simulink model "sim4"  (R2024a)
settings: Solver=FixedStepAuto  StartTime=0.0  StopTime=10.0  FixedStep=1  RelTol=1e-3
settings Model: Creator=alexe  LastModifiedBy=alexe

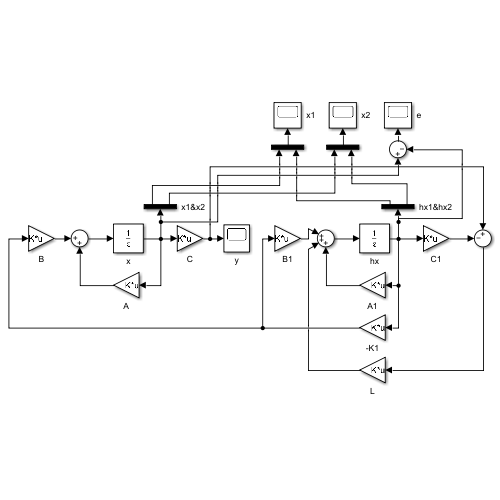
[thumbnail: Simulink's stored preview of the top-level diagram]
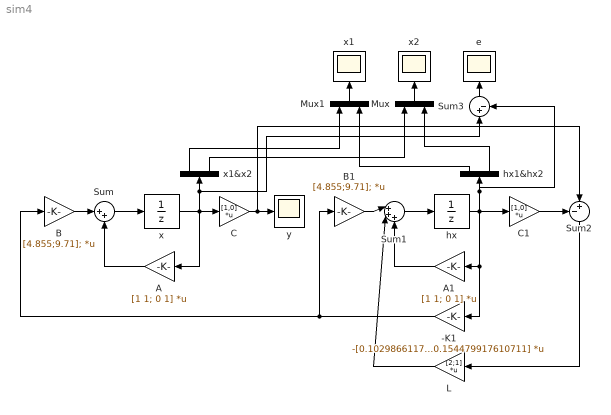
== system sim4 ==
  -K1 : Gain  Gain=-[0.102986611740474,0.154479917610711]  Multiplication=Matrix(K*u)
  A : Gain  Gain=[1 1; 0 1]  Multiplication=Matrix(K*u)
  A1 : Gain  Gain=[1 1; 0 1]  Multiplication=Matrix(K*u)
  B : Gain  Gain=[4.855;9.71];  Multiplication=Matrix(K*u)
  B1 : Gain  Gain=[4.855;9.71];  Multiplication=Matrix(K*u)
  C : Gain  Gain=[1,0]  Multiplication=Matrix(K*u)
  C1 : Gain  Gain=[1,0]  Multiplication=Matrix(K*u)
  L : Gain  Gain=[2;1]  Multiplication=Matrix(K*u)
  Mux : Mux  Inputs=2
  Mux1 : Mux  Inputs=2
  Sum : Sum  Inputs=|++
  Sum1 : Sum  Inputs=|+++
  Sum2 : Sum  Inputs=-+|
  Sum3 : Sum  Inputs=|+-
  e : Scope
  hx : UnitDelay  InitialCondition=[0;1];  SampleTime=-1  HasFrameUpgradeWarning=on
  hx1&hx2 : Demux  Outputs=2
  x : UnitDelay  InitialCondition=[1;0];  SampleTime=-1  HasFrameUpgradeWarning=on
  x1 : Scope
  x1&x2 : Demux  Outputs=2
  x2 : Scope
  y : Scope
  wires:
  Sum/1 -> x/1
  x/1 -> A/1, C/1, Sum3/1, x1&x2/1
  A/1 -> Sum/2
  B/1 -> Sum/1
  C/1 -> y/1, Sum2/2
  B1/1 -> Sum1/1
  hx/1 -> Sum3/2, hx1&hx2/1, C1/1, -K1/1, A1/1
  -K1/1 -> B1/1, B/1
  Sum1/1 -> hx/1
  C1/1 -> Sum2/1
  Sum2/1 -> L/1
  A1/1 -> Sum1/3
  L/1 -> Sum1/2
  Mux1/1 -> x1/1
  hx1&hx2/1 -> Mux1/2
  x1&x2/1 -> Mux1/1
  Mux/1 -> x2/1
  hx1&hx2/2 -> Mux/2
  x1&x2/2 -> Mux/1
  Sum3/1 -> e/1
